simulink model "MAS_direct_start"  (R2024b)
settings: Solver=VariableStepAuto  StartTime=0.0  StopTime=10  RelTol=1e-3
settings Model: Creator=firas  LastModifiedBy=firas

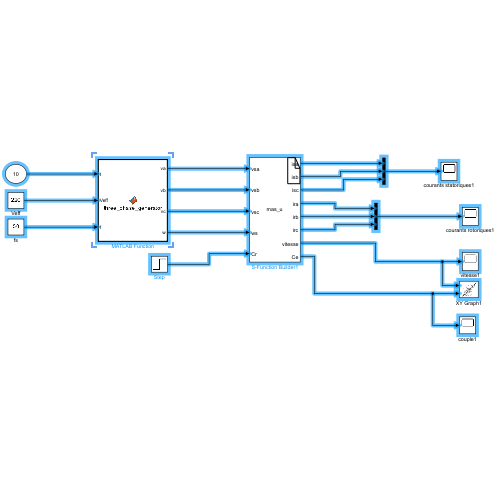
[thumbnail: Simulink's stored preview of the top-level diagram]
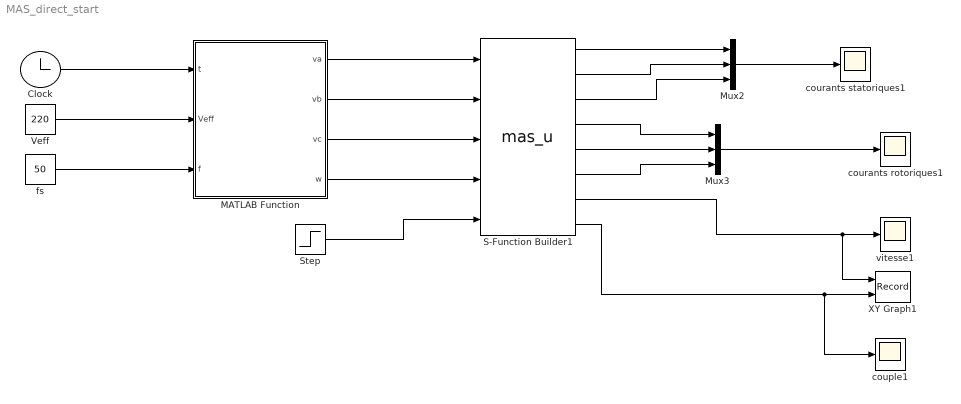
== system MAS_direct_start ==
  Clock : Clock
  MATLAB Function : MATLAB Function  TreatAsAtomicUnit=on
  Mux2 : Mux  Inputs=3
  Mux3 : Mux  Inputs=3
  S-Function Builder1 : S-Function  FunctionName=mas_u  SFunctionModules=mas_u_wrapper.c  SFunctionDeploymentMode=off  EnableBusSupport=off  mask(S-Function Builder){}
      mask help: Simulink:masks:SFunctionBuilder_MD
      mask init:
      | val = [[.9  0.75 0.75 1 1 .9 .9 1]',[1 1 0.75 0.75 .9 .9 1 .9]'];try , sys = get_param(gcb,'SfunBuilderFcnName');if isempty(sys), sys = get_param(gcb,'FunctionName'); end,catch, sys = get_param(gcb,'FunctionName'); end
      settings: CopyFcn=set_param(gcbh,'LinkStatus','none')  OpenFcn=sfunctionwizard(gcbh)
      mask Display:
      | plot(val(:,1),val(:,2))
      | disp(sys)
      | port_label('input',1,sprintf('%s', 'vsa'),'interpreter','tex')
      | port_label('input',2,sprintf('%s', 'vsb'),'interpreter','tex')
      | port_label('input',3,sprintf('%s', 'vsc'),'interpreter','tex')
      | port_label('input',4,sprintf('%s', 'ws'),'interpreter','tex')
      | port_label('input',5,sprintf('%s', 'Cr'),'interpreter','tex')
      | port_label('output',1,sprintf('%s', 'isa'),'interpreter','tex')
      | port_label('output',2,sprintf('%s', 'isb'),'interpreter','tex')
      | port_label('output',3,sprintf('%s', 'isc'),'interpreter','tex')
      | port_label('output',4,sprintf('%s', 'ira'),'interpreter','tex')
      | port_label('output',5,sprintf('%s', 'irb'),'interpreter','tex')
      | port_label('output',6,sprintf('%s', 'irc'),'interpreter','tex')
      | port_label('output',7,sprintf('%s', 'vitesse'),'interpreter','tex')
      | port_label('output',8,sprintf('%s', 'Ce'),'interpreter','tex')
  Step : Step  Time=5  After=10  SampleTime=0
  Veff : Constant  Value=220
  XY Graph1 : Record  FileSettingsInternal="{\"entries\":[{\"content\":{\"excelSettings\":{\"content\":{},\"type\":\"Streamout.ExcelSettings\"}},\"type\":\"Streamout.FileSettingStorage\",\"uuid\":\"\"}],\"packageUris\":[\"http:\\/\\/schema.mathworks.com\\/mf0\\/streamout_blocks\\/R2020a\"],\"version\":\"1.0\"}"  Layout=[1 1]  SignalsInternal="{\"entries\":[{\"content\":{\"signals\":[{\"content\":{\"blockPath\":[],\"dimensions\":[1],\"domain\":\"\",\"lineColor\":\"#a2142f\",\"plots\":[ 1 ],\"port\":1,\"sid\":[\"\"],\"signalID\":1,\"signalName\":\"S-Function Builder1:7\"},\"type\":\"RecordBlkView.Signal\",\"uuid\":\"\"},{\"content\":{\"blockPath\":[],\"dimensions\":[1],\"domain\":\"\",\"lineColor\":\"#139fff\",\"plots\":[ 1 ],\"port\":2,\"sid\":[\"\"],\"signalID\":2,\"signalName\":\"S-Function Builder1:8\"},\"type\":\"RecordBlkView.Signal\",\"uuid\":\"\"}]},\"type\":\"RecordBlkView.InputSignals\",\"uuid\":\"\"}],\"packageUris\":[\"http:\\/\\/schema.mathworks.com\\/mf0\\/streamout_blocks\\/R2020a\"],\"version\":\"1.0\"}"  VisualizationBindings="{\"xyplotplugin\":{\"info\":[{\"series\":[{\"bindingParametersList\":[{\"parameter\":\"X-Axis\",\"signalID\":1,\"signalName\":\"S-Function Builder1:7\"},{\"parameter\":\"Y-Axis\",\"signalID\":2,\"signalName\":\"S-Function Builder1:8\"}],\"seriesID\":0}],\"subplotID\":1}]}}"  CompatibilityTag=XY
  couple1 : Scope
  courants rotoriques1 : Scope
  courants statoriques1 : Scope
  fs : Constant  Value=50
  vitesse1 : Scope
  wires:
  Step/1 -> S-Function Builder1/5
  fs/1 -> MATLAB Function/3(f)
  Veff/1 -> MATLAB Function/2(Veff)
  Clock/1 -> MATLAB Function/1(t)
  S-Function Builder1/1 -> Mux2/1
  S-Function Builder1/2 -> Mux2/2
  S-Function Builder1/3 -> Mux2/3
  S-Function Builder1/4 -> Mux3/1
  S-Function Builder1/5 -> Mux3/2
  S-Function Builder1/6 -> Mux3/3
  S-Function Builder1/7 -> XY Graph1/1, vitesse1/1
  S-Function Builder1/8 -> couple1/1, XY Graph1/2
  Mux2/1 -> courants statoriques1/1
  Mux3/1 -> courants rotoriques1/1
  MATLAB Function/1(va) -> S-Function Builder1/1
  MATLAB Function/2(vb) -> S-Function Builder1/2
  MATLAB Function/3(vc) -> S-Function Builder1/3
  MATLAB Function/4(w) -> S-Function Builder1/4

== matlab function MAS_direct_start/MATLAB Function ==
  data: t input; Veff input; va output; f input; vb output; vc output; w output
function [va,vb,vc,w] = three_phase_generator(t,Veff,f)

Vm = sqrt(2)*Veff;

w = 2*pi*f;

va = Vm*cos(w*t);

vb = Vm*cos(w*t - 2*pi/3);

vc = Vm*cos(w*t + 2*pi/3);
